simulink model "obieg_pierwotny"  (R2016a)
settings: Solver=VariableStepAuto  StartTime=0.0  StopTime=10.0  RelTol=1e-3
values from neighbouring files (symbols this model uses):
  c_psi = 13.75 * (10 ^ 6)    (= 13750000)    [unit_1.m]
  K_T_SG = 9.5296*(10^6)    (= 9529600)    [unit_1.m]
  m_in = 1.4222    [unit_1.m]
  m_out = 2.9722    [unit_1.m]
  N = 99.3    [Unit_3.m]    (also in unit_1.m = 100.3; unit_4.m = 100.8)
  T_PC_I = 246.1    [unit_1.m]
  T_SG = 255.13    [unit_1.m]
  W_loss_PC = 2.2469 * (10 ^ 8)    (= 224690000)    [unit_1.m]
undefined symbols (not defined in the file or in its folder): C_p_PC
settings Model: Creator=Michal Chruscinski  LastModifiedBy=Michal Chruscinski
settings GRTTargetCC: GeneratePreprocessorConditionals=Use local settings

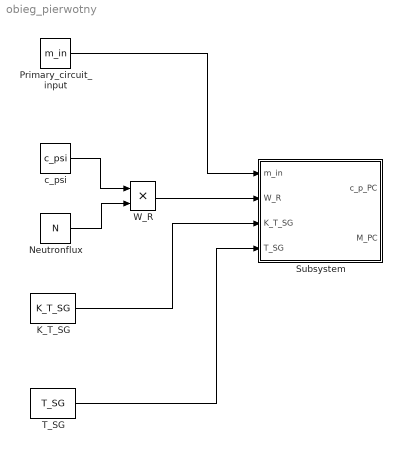
== system obieg_pierwotny ==
  K_T_SG : Constant  Value=K_T_SG
  Neutronflux : Constant  Value=N
  Primary_circuit_input : Constant  Value=m_in
  Subsystem : Subsystem
  T_SG : Constant  Value=T_SG
  W_R : Product
  c_psi : Constant  Value=c_psi
  wires:
  c_psi/1 -> W_R/1
  Neutronflux/1 -> W_R/2
  W_R/1 -> Subsystem/2(W_R)
  Primary_circuit_input/1 -> Subsystem/1(m_in)
  K_T_SG/1 -> Subsystem/3(K_T_SG)
  T_SG/1 -> Subsystem/4(T_SG)

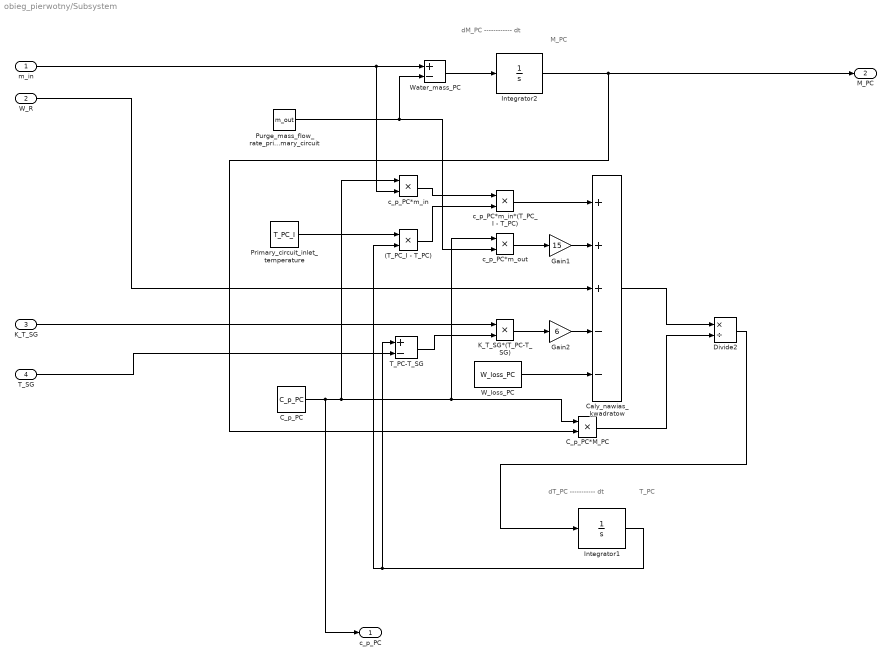
== system obieg_pierwotny/Subsystem ==
  note: dM_PC
      | ------------
      |      dt
  note: M_PC
  note: dT_PC
      | -----------
      |     dt
  note: T_PC
  m_in : Inport
  W_R : Inport  Port=2
  K_T_SG : Inport  Port=3
  T_SG : Inport  Port=4
  (T_PC_I - T_PC) : Product
  C_p_PC : Constant  Value=C_p_PC
  C_p_PC*M_PC : Product
  Caly_nawias_kwadratow : Sum  Inputs=+++--
  Divide2 : Product  Inputs=*/
  Gain1 : Gain  Gain=15
  Gain2 : Gain  Gain=6
  Integrator1 : Integrator
  Integrator2 : Integrator
  K_T_SG*(T_PC-T_SG) : Product
  Primary_circuit_inlet_temperature : Constant  Value=T_PC_I
  "Purge_mass_flow_rate_primary_circuit " : Constant  Value=m_out
  T_PC-T_SG : Sum  Inputs=+-
  W_loss_PC : Constant  Value=W_loss_PC
  Water_mass_PC : Sum  Inputs=+-
  c_p_PC*m_in : Product
  c_p_PC*m_in*(T_PC_I - T_PC) : Product
  c_p_PC*m_out : Product
  c_p_PC : Outport
  M_PC : Outport  Port=2
  wires:
  m_in/1 -> c_p_PC*m_in/2, Water_mass_PC/1
  "Purge_mass_flow_rate_primary_circuit "/1 -> c_p_PC*m_out/2, Water_mass_PC/2
  Water_mass_PC/1 -> Integrator2/1
  Integrator1/1 -> T_PC-T_SG/1, (T_PC_I - T_PC)/2
  Integrator2/1 -> C_p_PC*M_PC/2, M_PC/1
  C_p_PC/1 -> c_p_PC/1, C_p_PC*M_PC/1, c_p_PC*m_out/1, c_p_PC*m_in/1
  C_p_PC*M_PC/1 -> Divide2/2
  Divide2/1 -> Integrator1/1
  Caly_nawias_kwadratow/1 -> Divide2/1
  c_p_PC*m_in*(T_PC_I - T_PC)/1 -> Caly_nawias_kwadratow/1
  c_p_PC*m_in/1 -> c_p_PC*m_in*(T_PC_I - T_PC)/1
  (T_PC_I - T_PC)/1 -> c_p_PC*m_in*(T_PC_I - T_PC)/2
  Primary_circuit_inlet_temperature/1 -> (T_PC_I - T_PC)/1
  c_p_PC*m_out/1 -> Gain1/1
  Gain1/1 -> Caly_nawias_kwadratow/2
  Gain2/1 -> Caly_nawias_kwadratow/4
  K_T_SG*(T_PC-T_SG)/1 -> Gain2/1
  T_PC-T_SG/1 -> K_T_SG*(T_PC-T_SG)/2
  K_T_SG/1 -> K_T_SG*(T_PC-T_SG)/1
  T_SG/1 -> T_PC-T_SG/2
  W_loss_PC/1 -> Caly_nawias_kwadratow/5
  W_R/1 -> Caly_nawias_kwadratow/3
